simulink model "SFM_simulink_16kfs_2017a"  (R2017a)
settings: Solver=FixedStepDiscrete  StartTime=0.0  StopTime=inf  RelTol=1e-3
libraries: audiosources x1, dspsnks4 x1, dspxfrm3 x1, dspvision x1, simulink x1, dspsigops x1
settings Model: Creator=zhouyiliang  LastModifiedBy=zhouyiliang
settings SolverCC: AutoInsertRateTranBlk=on
settings DataIOCC: LimitDataPoints=on  SaveOutput=off  SignalLogging=off  SaveTime=off  ReturnWorkspaceOutputs=on
settings OptimizationCC: LifeSpan=inf
settings DebuggingCC: AlgebraicLoopMsg=error  SingleTaskRateTransMsg=error  AllowSymbolicDim=off  SFUnexpectedBacktrackingDiag=warning  SFNoUnconditionalDefaultTransitionDiag=warning  SFExecutionAtInitializationDiag=none
settings GRTTargetCC: TargetLangStandard=C89/C90 (ANSI)
settings ConfigComp: CovMetricSettings=dw  CovSaveCumulativeToWorkspaceVar=on  CovSaveSingleToWorkspaceVar=on  CovExternalEMLEnable=off  CovSFcnEnable=off

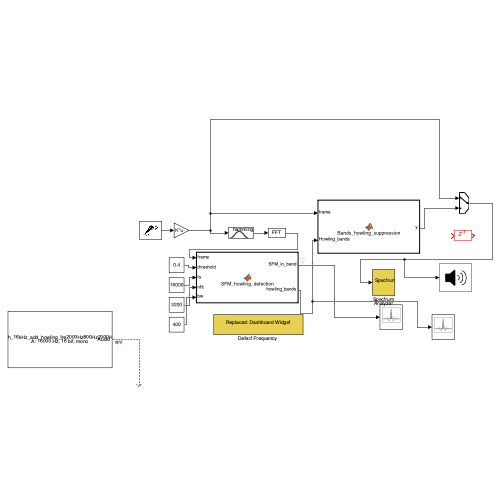
[thumbnail: Simulink's stored preview of the top-level diagram]
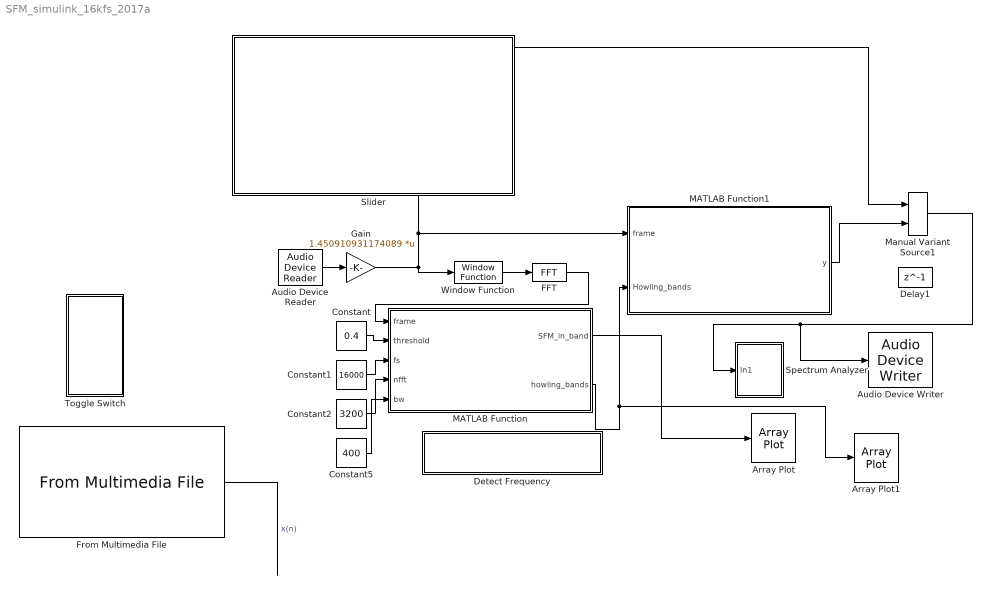
== system SFM_simulink_16kfs_2017a ==
  Array Plot : ArrayPlot  DefaultConfigurationName=dsp.scopes.ArrayPlotBlockSpecification
  Array Plot1 : ArrayPlot  DefaultConfigurationName=dsp.scopes.ArrayPlotBlockSpecification
  Audio Device Reader : audiosources/Audio Device Reader  Driver=CoreAudio  Device=External Microphone  SampleRate=16000  NumChannels=1  SamplesPerFrame=1600  BitDepth=16-bit integer  NumBuffers=10  DefaultInputChannelMapping=on  InputChannelMapping=1:2  OutputNumOverrunSamples=off  OutputDataType=double  DriverIdx=5  DeviceWarnFlag=''
  Audio Device Writer : dspsnks4/Audio Device Writer  Driver=CoreAudio  Device=External Headphones  InheritSampleRate=on  SampleRate=44100  BitDepth=16-bit integer  BufferSize=4096  NumBuffers=10  DefaultOutputChannelMapping=on  OutputChannelMapping=1:2  OutputNumUnderrunSamples=off  DriverIdx=5  DeviceWarnFlag=''
  Constant : Constant  Value=0.4
  Constant1 : Constant  Value=16000
  Constant2 : Constant  Value=3200
  Constant5 : Constant  Value=400
  Delay1 : Delay  DelayLength=1  InitialCondition=0
  "Detect Frequency " : Subsystem  Description=Replaced Block  mask(Replaced Block){}
      mask help: This block has been replaced with an empty subsystem because it used functionality that is unavailable in Simulink R2017a.
      mask Display: fprintf('Replaced: %s\n','Dashboard Widget')
  FFT : dspxfrm3/FFT  FFTImplementation=Auto  CompMethod=Table lookup  TableOpt=NEW  TableOptActive=Speed  BitRevOrder=off  Normalize=off  InheritFFTLength=off  FFTLength=3200  WrapInput=on  roundingMode=Floor  overflowMode=off  firstCoeffDataTypeStr=Inherit: Same word length as input  firstCoeffLastDataTypeStr=Inherit: Same word length as input  outputMin=[]  outputMax=[]
  From Multimedia File : dspvision/From Multimedia File  inputFilename=/Users/zhouyiliang/Desktop/work/sound_output/speech_16kHz_add_howling_tre2000Hz800Hz2000Hz.wav  loop=on  numPlays=inf  outputStreams=Audio only  videoDataType=single  audioDataType=double  inheritSampleTime=on  userDefinedSampleTime=1/30  noAudioOutput=off  isIntensityVideo=off  fourcc=RGB  colorVideoFormat=Separate color signals  outputEOF=off  dataOrg=Column-major  audioFrameSize=800  computeAudioFrameSize=off  outSamplingMode=Sample based
  Gain : Gain  Gain=1.450910931174089  Multiplication=Matrix(K*u)
  MATLAB Function : MATLAB Function  TreatAsAtomicUnit=on
  MATLAB Function1 : MATLAB Function  TreatAsAtomicUnit=on
  Manual Variant Source1 : simulink/Signal Routing/Manual Variant Source  NumChoices=2  OverrideUsingVariant=V_1
  Slider : Subsystem  DialogController=hmiCreateDDGDialog  IsWebBlock=on  mask(MWDashboardBlock){webBlockId=42ae5c65-603c-4e59-b7e2-6c9542fb2d6f, webBlockType=slider, ShowInLibBrowser=on, ShowInitialText=on, HMISrcModelName=SFM_simulink_16kfs_2017a}
      mask prompts: webBlockId "WebBlock Id"; webBlockType "WebBlock Type"; HMISrcModelName "Source Model"
      mask help: Set value to tune parameters or variables.
      mask Help: helpview([docroot '/mapfiles/simulink.map'], 'hmi_slider')
      mask Display:
      | if strcmp(get_param(bdroot(gcb),'BlockDiagramType'),'library')
      |  image([(matlabroot) '/toolbox/simulink/hmi/icons/Slider.png'])
      | end
  Spectrum Analyzer : Subsystem  Description=Replaced Block  mask(Replaced Block){}
      mask help: This block has been replaced with an empty subsystem because it used functionality that is unavailable in Simulink R2017a.
      mask Display: fprintf('Replaced: %s\n','SpectrumAnalyzer')
  Toggle Switch : Subsystem  DialogController=hmiCreateDDGDialog  IsWebBlock=on  mask(MWDashboardBlock){webBlockId=d06d4e76-ac2f-434b-a177-6adf76c4a06e, webBlockType=toggleswitch, ShowInLibBrowser=on, ShowInitialText=on, HMISrcModelName=SFM_simulink_16kfs_2017a}
      mask prompts: webBlockId "WebBlock Id"; webBlockType "WebBlock Type"; HMISrcModelName "Source Model"
      mask help: Set on/off value to tune parameters or variables.
      mask Help: helpview([docroot '/mapfiles/simulink.map'], 'hmi_switch')
      mask Display:
      | if strcmp(get_param(bdroot(gcb),'BlockDiagramType'),'library')
      |  image([(matlabroot) '/toolbox/simulink/hmi/icons/ToggleSwitch.png'])
      | end
  Window Function : dspsigops/Window Function  winmode=Apply window to input  wintype=Hamming  sampmode=Continuous  samptime=1  N=64  Rs=50  beta=10  winsamp=Symmetric  UserWindow=hamming  OptParams=off  UserParams={'symmetric'}  dataType=double  isSigned=on  wordLen=16  udDataType=sfix(16)  fracBitsMode=Best precision  numFracBits=15  roundingMode=Floor  overflowMode=off  numSidelobes=4  sidelobeLevel=-30
  wires:
  FFT/1 -> MATLAB Function/1(frame)
  Constant/1 -> MATLAB Function/2(threshold)
  Constant1/1 -> MATLAB Function/3(fs)
  Constant2/1 -> MATLAB Function/4(nfft)
  Constant5/1 -> MATLAB Function/5(bw)
  Window Function/1 -> FFT/1
  Audio Device Reader/1 -> Gain/1
  From Multimedia File/1 -> ?  "x(n)"
  MATLAB Function1/1(y) -> Manual Variant Source1/2
  Manual Variant Source1/1 -> Audio Device Writer/1, Spectrum Analyzer/1(In1)
  MATLAB Function/1(SFM_in_band) -> Array Plot/1
  MATLAB Function/2(howling_bands) -> Array Plot1/1, MATLAB Function1/2(Howling_bands)
  Gain/1 -> Window Function/1, MATLAB Function1/1(frame), Manual Variant Source1/1

== system SFM_simulink_16kfs_2017a/Detect Frequency  ==

== system SFM_simulink_16kfs_2017a/Slider ==

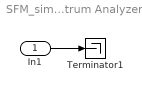
== system SFM_simulink_16kfs_2017a/Spectrum Analyzer ==
  In1 : Inport
  Terminator1 : Terminator
  wires:
  In1/1 -> Terminator1/1

== system SFM_simulink_16kfs_2017a/Toggle Switch ==

== matlab function SFM_simulink_16kfs_2017a/MATLAB Function1 ==
  data: frame input; Howling_bands input size=[20 1]; y output
%% EQ

function y = Bands_howling_suppression(frame, Howling_bands)
% Suppress howling noise in signal by attenuating frequency bands
% specified in SFM_in_band.
fs = 16000;  % Sampling frequency in Hz
nfft = 3200;  % FFT length
% frame = fft(signal, nfft);  % Compute spectrum of signal

f_center = [36.1767908943890	47.7165473068120	62.9372819034748	83.0131616172483	109.492891864320	144.419187695662	190.486354132649	251.248131842519	331.391841907987	437.099977929402	576.527139611757	760.429099730129	1002.99253233036	1322.92940954980	1744.92049166657	2301.51926494252	3035.66320196194	4003.98606959998	5281.18680464596	6965.79198347538];
% bw_vector = [10.0479428386143	13.2530588795051	17.4805502464275	23.0565365849553	30.4111639393061	40.1117873335244	52.9067380091402	69.7830516375018	92.0426108107617	121.402575640709	160.127849942245	211.205801786369	278.576716819166	367.437762113383	484.643909112229	639.236743900871	843.141958601118	1112.08933018402	1466.82615625138	1934.71775536878];
bw_vector = [30	30	40	50	100	150	300 400	500	600	800	900	1000	1000	1200	1400	1600	1800	2000	2000];
f_lower = f_center - bw_vector/2;
f_upper = f_center + bw_vector/2;
% f_lower = [31.1528194750819	41.0900178670594	54.1970067802611	71.4848933247707	94.2873098946670	124.363294028899	164.032985128079	216.356606023768	285.370536502607	376.398690109047	496.463214640634	654.826198836944	863.704173920776	1139.21052849311	1502.59853711045	1981.90089299208	2614.09222266138	3447.94140450797	4547.77372652027	5998.43310579098];
% f_upper = [41.2007623136961	54.3430767465645	71.6775570266885	94.5414299097260	124.698473833973	164.475081362424	216.939723137219	286.139657661270	377.413147313368	497.801265749757	656.591064582880	866.032000623313	1142.28089073994	1506.64829060649	1987.24244622268	2621.13763689295	3457.23418126250	4560.03073469199	6014.59988277165	7933.15086115977];

idx_lower = round(f_lower/(fs/nfft)) + 1;
idx_upper = round(f_upper/(fs/nfft)) + 1;

% Attenuate frequency bands with howling
for b = 1:size(Howling_bands, 1)
    if Howling_bands(b) == 0
        idx = idx_lower(b):idx_upper(b);
        if any(idx)
            frame(idx) = frame(idx) .* 0.01;  % Attenuate by a factor of 10
        end
    end
end

output = real(ifft(frame, nfft));
y = output(1:1600);  % Truncate to original signal length
end


%%%%%%%%%%%%%%%%%%%%%%%%%%%%%%%%%%%%%%%%%%%%%%%%%%%%%%%
%% notch filter
% function y = Bands_howling_suppression(signal, SFM_in_band)
% % Suppress howling noise in the specified frequency bands using a notch filter.
% % Args:
% %   - signal: Original audio signal with howling noise.
% %   - SFM_in_band: A binary vector of length nfft/2bw, where 1 indicates howling
% %     in the corresponding frequency band, and 0 indicates no howling.
% % Returns:
% %   - output: The denoised signal with howling suppression.
% 
% % Set filter parameters
% fs = 16000;
% f_bw = 10; % bandwidth of notch filter
% Q = 10; % quality factor of notch filter
% 
% % Create a bandpass filter for each band
% f_center = [36.1767908943890	47.7165473068120	62.9372819034748	83.0131616172483	109.492891864320	144.419187695662	190.486354132649	251.248131842519	331.391841907987	437.099977929402	576.527139611757	760.429099730129	1002.99253233036	1322.92940954980	1744.92049166657	2301.51926494252	3035.66320196194	4003.98606959998	5281.18680464596	6965.79198347538];
% % bw_vector = [10.0479428386143	13.2530588795051	17.4805502464275	23.0565365849553	30.4111639393061	40.1117873335244	52.9067380091402	69.7830516375018	92.0426108107617	121.402575640709	160.127849942245	211.205801786369	278.576716819166	367.437762113383	484.643909112229	639.236743900871	843.141958601118	1112.08933018402	1466.82615625138	1934.71775536878];
% bw_vector = [30	30	40	50	100	150	300 400	500	600	800	900	1000	1000	1200	1400	1600	1800	2000	2000];
% f_lower = f_center - bw_vector/2;
% f_upper = f_center + bw_vector/2;
% % f_center = linspace(fs/(2*length(SFM_in_band)), fs/2, length(SFM_in_band)).';
% % f_lower = f_center - f_bw/2;
% % f_upper = f_center + f_bw/2;
% 
% b=zeros(20,3);
% a=zeros(20,3);
% % Create a notch filter for each howling band
% for i = 1:length(SFM_in_band)
%     if SFM_in_band(i) == 1
%         % Calculate the center frequency of the howling band
%         f_center = (i-1)*fs/length(SFM_in_band);
%         % Create a notch filter
%         wo = f_center/(fs/2);
%         bw = wo/Q;
%         [b_notch,a_notch] = iirnotch(wo,bw);
%         % Apply the notch filter to the corresponding bandpass filter
%         [b_n,a_n] = butter(2, [f_lower(i)./fs f_upper(i)./fs]);
%         [b(i,:),a(i,:)] = sosfilt(b_notch,a_notch,b_n,a_n);
%     end
% end
% 
% % Apply the bandpass filters to the signal
% output = zeros(size(signal));
% for i = 1:length(SFM_in_band)
%     y = filter(b(i,:), a(i,:), signal);
%     output = output + y;
% end
% y = output(1:800);  % Truncate to original signal length
% end

== matlab function SFM_simulink_16kfs_2017a/MATLAB Function ==
  data: frame input; threshold input; fs input; nfft input; bw input; SFM_in_band output size=[20 1]; howling_bands output size=[20 1]
function [SFM_in_band,howling_bands] = SFM_howling_detection(frame,threshold,fs,nfft,bw)
% Args:
%   - frame: Spectrum of one frame. The frequency range should be between
%     0 and fs/2 Hz, with a total of nfft/2 frequency bins.
%   - threshold: SFM threshold value for howling detection.
%   - fs: Sampling frequency in Hz.
%   - nfft: FFT length.
%   - bw: Bandwidth of each frequency band in Hz.

% Returns:
%   - SFM_in_band: A binary vector of length nfft/2bw, where 1 indicates howling
%     in the corresponding frequency band, and 0 indicates no howling.
%       (1-20 array) eg.0 0 1 0 0 means the 3rd band is howling 
%   - howling_bands: A vector containing the indices of the frequency bands with
%     howling noise, or an empty array if no howling is detected.

%%%%%%%%%%%%%1111111111111111111111111111111111111111111111111111111111       
%%%%%%Function: compute the spectral flatness measure(SFM) result 
%         %SFM (n, b) = product^(1/w) /  [sum*(1/w)]
% % Compute frequency indices for each band
% frame = abs(frame);
% f_center = linspace(bw/2, fs/2-bw/2, fs/(2*bw)).';
% f_lower = f_center - bw/2;
% f_upper = f_center + bw/2;
% idx_lower = round(f_lower/(fs/nfft)) + 1;
% idx_upper = round(f_upper/(fs/nfft)) + 1;
% 
% % Initialize SFM values to 1 (for non-empty bands)
% SFM_in_band = ones(fs/(2*bw), 1);
% howling_bands =  ones(fs/(2*bw), 1);
% w = bw/fs*nfft;
% % Compute SFM for each band
% for b = 1:fs/(2*bw)
%     idx = idx_lower(b):idx_upper(b);
%     if any(idx)
%         numerator = prod(frame(idx)).^(1/w);
%         denominator = sum(frame(idx))./w;
%         SFM_in_band(b) = numerator/denominator;
% %%%%%%%%%% Howling in bands is marked by a flag updated as %%%%%%%%%%
%         if SFM_in_band(b) < threshold
%             howling_bands(b) = 0;
%         end
%     end
% end
% 
% % Mark bands with SFM below threshold as howling
%  % Mark howling in a band with a flag
% 
% 
% end

%%%%%%%%%%%%%22222222222222222222222222222222222222222222222222 
%%%%%%Function: compute the spectral flatness measure(SFM) result 
%% with 20 1/3 octave bands, variable bw 
frame = abs(frame);

f_center = [36.1767908943890	47.7165473068120	62.9372819034748	83.0131616172483	109.492891864320	144.419187695662	190.486354132649	251.248131842519	331.391841907987	437.099977929402	576.527139611757	760.429099730129	1002.99253233036	1322.92940954980	1744.92049166657	2301.51926494252	3035.66320196194	4003.98606959998	5281.18680464596	6965.79198347538];
% bw_vector = [10.0479428386143	13.2530588795051	17.4805502464275	23.0565365849553	30.4111639393061	40.1117873335244	52.9067380091402	69.7830516375018	92.0426108107617	121.402575640709	160.127849942245	211.205801786369	278.576716819166	367.437762113383	484.643909112229	639.236743900871	843.141958601118	1112.08933018402	1466.82615625138	1934.71775536878];
bw_vector = [30	30	40	50	100	150	300 400	500	600	800	900	1000	1000	1200	1400	1600	1800	2000	2000];
f_lower = f_center - bw_vector/2;
f_upper = f_center + bw_vector/2;
idx_lower = round(f_lower/(fs/nfft)) + 1;
idx_upper = round(f_upper/(fs/nfft)) + 1;

% Initialize SFM values to 1 (for non-empty bands)
SFM_in_band = ones(20, 1);
howling_bands =  ones(20, 1);
bw_vector = bw_vector/fs*nfft;
% Compute SFM for each band
for b = 1:20
    idx = idx_lower(b):idx_upper(b);
    if any(idx)
        numerator = prod(frame(idx)).^(1/bw_vector(b));
        denominator = sum(frame(idx))./bw_vector(b);
        SFM_in_band(b) = numerator/denominator;
%%%%%%%%%% Howling in bands is marked by a flag updated as %%%%%%%%%%
        if SFM_in_band(b) < threshold
            howling_bands(b) = 0;
        end
    end
end

% Mark bands with SFM below threshold as howling
 % Mark howling in a band with a flag

end





%%%%%%%%%%%%%333333333333333333333333333333333333333333333333333
%% original 
% %%%%%%%%%%% cut spectrum into 20 bands  %%%%%%%%%%%
% frame = abs(frame);
% f_all = linspace(0, fs, nfft);
% f_center = (linspace(200,7800,20))';
% f_lower_upper = [(f_center-200) (f_center+200)];
% counter=1;
% SFM_in_band = ones(fs/(2*bw), 1);
% howling_bands =  ones(fs/(2*bw), 1);
% w = bw/fs*nfft;
% for b = 1:20 % loop for 20 bands
%     indexes = find(f_all >= f_lower_upper(b,1) & f_all< f_lower_upper(b,2));
%     if isempty(indexes) 
%         SFM_in_band(b) = 1; % default value is 1, if howling value should be smaller
%         counter=counter+1;
%     else
%         numerator = (prod(frame(indexes)))^(1/w); % product of all spectrums in the band
%         denominator = (1/w) * sum(frame( indexes ));% sum of all spectrums in the band
%         SFM_in_band(b) = numerator/denominator;
% %%%%%%%%%% Howling in bands is marked by a flag updated as %%%%%%%%%%
%         if SFM_in_band(b) < threshold
%             howling_bands(b) = 0;
%         end
%     end
% end
% 
% % Mark bands with SFM below threshold as howling
%  % Mark howling in a band with a flag
% 
% 
% end
